simulink model "TestTraj"  (R2013b)
settings: Solver=FixedStepDiscrete  StartTime=0.0  StopTime=5  FixedStep=Ts  RelTol=1e-3
settings Model: Creator=LukePH  LastModifiedBy=LukePH

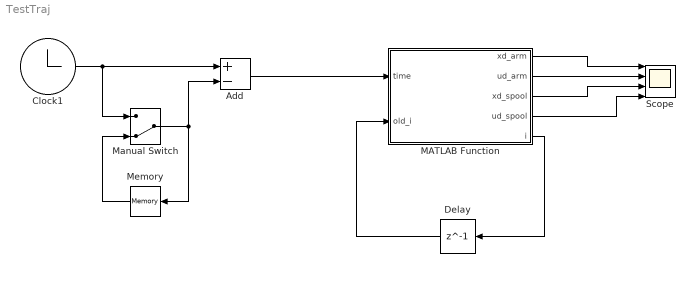
== system TestTraj ==
  Add : Sum  Inputs=+-
  Clock1 : Clock
      settings: Decimation=5
  Delay : Delay  DelayLength=1  InitialCondition=1
  MATLAB Function : MATLAB Function  TreatAsAtomicUnit=on
  Manual Switch : ManualSwitch  CurrentSetting=0
  Memory : Memory  InheritSampleTime=on
  Scope : Scope  NumInputPorts=4
      settings: YMin=-5~-5~-5~-5  YMax=5~5~5~5
  wires:
  Delay/1 -> MATLAB Function/2(old_i)
  MATLAB Function/5(i) -> Delay/1
  Clock1/1 -> Add/1, Manual Switch/1
  Manual Switch/1 -> Memory/1, Add/2
  Memory/1 -> Manual Switch/2
  Add/1 -> MATLAB Function/1(time)
  MATLAB Function/2(ud_arm) -> Scope/2
  MATLAB Function/1(xd_arm) -> Scope/1
  MATLAB Function/3(xd_spool) -> Scope/3
  MATLAB Function/4(ud_spool) -> Scope/4

== matlab function TestTraj/MATLAB Function ==
  data: time input; xd_arm output; ud_arm output; xd_spool output; ud_spool output; old_i input; i output
function [xd_arm, ud_arm, xd_spool, ud_spool, i] = TrajectoryTimeMap(time,old_i)
%#codegen

% Load Data
D = load('CastingTrajectory.mat');

accu = 10^6;        % Accuracy

if time > max(D.Time) % Check to see if end of simulation
    xd_arm   = D.xd_arm(end);
    ud_arm   = D.ud_arm(end);
    xd_spool = D.xd_spool(end);
    ud_spool = D.ud_spool(end);
    i = old_i;
else % Find closest time
    [Val, I] = min(round(accu*abs(D.Time - time))/accu);
    xd_arm   = D.xd_arm(I);
    ud_arm   = D.ud_arm(I);
    xd_spool = D.xd_spool(I);
    ud_spool = D.ud_spool(I);
    i = I;
end %If
end % Function
